simulink model "SF011A_EotLrng"  (R2013b)
settings: Solver=FixedStepDiscrete  SolverMode=SingleTasking  StartTime=0.0  StopTime=1  FixedStep=0.002  RelTol=1e-3
values from neighbouring files (symbols this model uses):
  ARCHGLBPRM_FLOATZEROTHD_ULS_F32 = DataDict.Constant    [SF011A_EotLrng_DataDict.m]
  CNVTOMILLISEC_MILLISECPERCNT_F32 = DataDict.Constant    [SF011A_EotLrng_DataDict.m]
  CORRLNFLT_CNT_U08 = DataDict.Constant    [SF011A_EotLrng_DataDict.m]
  DEBSTEP_CNT_U16 = DataDict.Constant    [SF011A_EotLrng_DataDict.m]
  EOTLIMDETD_CNT_LOGL = DataDict.Constant    [SF011A_EotLrng_DataDict.m]
  EOTLIMNOTDETD_CNT_LOGL = DataDict.Constant    [SF011A_EotLrng_DataDict.m]
  EotLrngAuthyStrtLrn = DataDict.Calibration    [SF011A_EotLrng_DataDict.m]
  EotLrngEotLrnTmr = DataDict.Calibration    [SF011A_EotLrng_DataDict.m]
  EotLrngHwAgOverTrvlCnt = DataDict.Calibration    [SF011A_EotLrng_DataDict.m]
  EotLrngHwAgOverTrvlEntr = DataDict.Calibration    [SF011A_EotLrng_DataDict.m]
  EotLrngHwAgOverTrvlExit = DataDict.Calibration    [SF011A_EotLrng_DataDict.m]
  EotLrngHwTqEotLrn = DataDict.Calibration    [SF011A_EotLrng_DataDict.m]
  EotLrngMotVelEotLrn = DataDict.Calibration    [SF011A_EotLrng_DataDict.m]
  EotLrngRackTrvlMax = DataDict.Calibration    [SF011A_EotLrng_DataDict.m]
  EotLrngRackTrvlMin = DataDict.Calibration    [SF011A_EotLrng_DataDict.m]
  EotLrngRstAuthyMin = DataDict.Calibration    [SF011A_EotLrng_DataDict.m]
  EotProtnRackTrvlLimrEna = DataDict.ImprtdCal    [SF011A_EotLrng_DataDict.m]
  HwAgOverTrvl = DataDict.NTC    [SF011A_EotLrng_DataDict.m]
  HWAGOVERTRVLMAXCNT_CNT_U08 = DataDict.Constant    [SF011A_EotLrng_DataDict.m]
  NODEBSTEP_CNT_U16 = DataDict.Constant    [SF011A_EotLrng_DataDict.m]
  OUTOFRNGFLT_CNT_U08 = DataDict.Constant    [SF011A_EotLrng_DataDict.m]
  RackEotStorgFlt = DataDict.NTC    [SF011A_EotLrng_DataDict.m]
  SIGAVLFLT_CNT_U08 = DataDict.Constant    [SF011A_EotLrng_DataDict.m]
undefined symbols (not defined in the file or in its folder): NtcSts1, NvmGetErrSts1, SigQlfr1
libraries: simulink x19, NxtrNvM x12, NxtrAbslt x5, NxtrLim x4, NxtrMax x3, NxtrMin x3
(part 5 of 7)

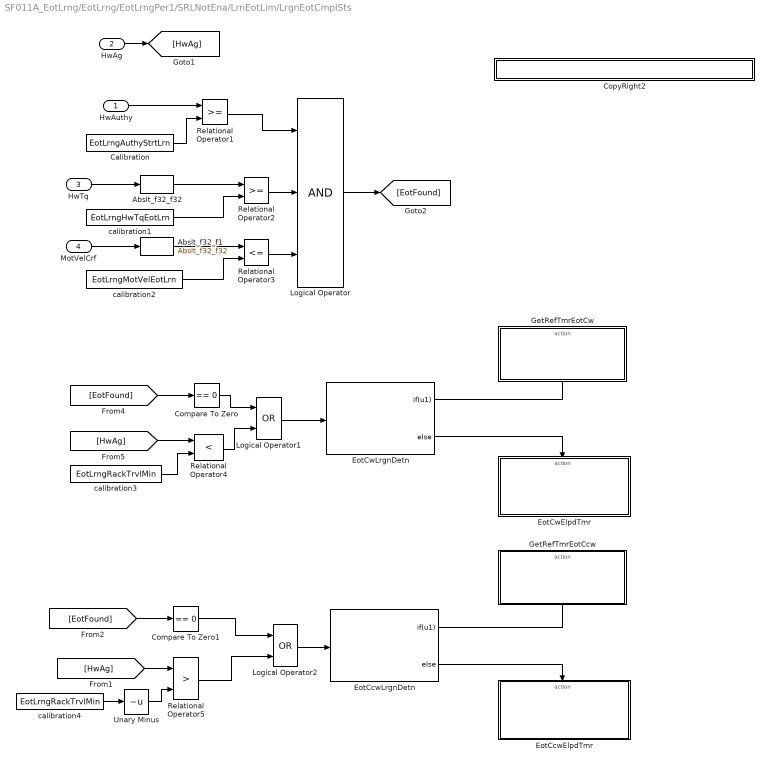
== system SF011A_EotLrng/EotLrng/EotLrngPer1/SRLNotEna/LrnEotLim/LrgnEotCmplSts ==
  HwAuthy : Inport  RequirementInfo="{'linktype_rmi_doors' '0000ba59 (/E-STEER Core/SubSystem Specifications/Application Functions/SF011A Learned EOT Limits)' '#SF011A_137' 'true' 'REQ:  SF011A_137' '' } %GIDa_6ae0917b_799c_4329_b7fc_536c1224b2ae"
  HwAg : Inport  Port=2
  HwTq : Inport  RequirementInfo="{'linktype_rmi_doors' '0000ba59 (/E-STEER Core/SubSystem Specifications/Application Functions/SF011A Learned EOT Limits)' '#SF011A_137' 'true' 'REQ:  SF011A_137' '' } %GIDa_43c992ac_a84d_4c9e_9654_d89dfe1e7ad2"  Port=3
  MotVelCrf : Inport  RequirementInfo="{'linktype_rmi_doors' '0000ba59 (/E-STEER Core/SubSystem Specifications/Application Functions/SF011A Learned EOT Limits)' '#SF011A_137' 'true' 'REQ:  SF011A_137' '' } %GIDa_06bf4615_f553_4b50_9b08_e34adfc1d38a"  Port=4
  Abslt_f32_f1 : NxtrAbslt/Abslt_f32_f32  RequirementInfo="{'linktype_rmi_doors' '0000ba59 (/E-STEER Core/SubSystem Specifications/Application Functions/SF011A Learned EOT Limits)' '#SF011A_137' 'true' 'REQ:  SF011A_137' '' } %GIDa_90d1ac47_d6a5_44ab_bd7c_cda08348b83e"  SFunctionSpec=single y1 = Abslt_f32_f32(single u1)
      settings: AttributesFormatString=%<Name>
  Abslt_f32_f32 : NxtrAbslt/Abslt_f32_f32  RequirementInfo="{'linktype_rmi_doors' '0000ba59 (/E-STEER Core/SubSystem Specifications/Application Functions/SF011A Learned EOT Limits)' '#SF011A_137' 'true' 'REQ:  SF011A_137' '' } %GIDa_6c8d8a4e_2031_40e8_8a2c_4552045f0482"  SFunctionSpec=single y1 = Abslt_f32_f32(single u1)
      settings: AttributesFormatString=%<Name>
  Calibration : Constant  RequirementInfo="{'linktype_rmi_doors' '0000ba59 (/E-STEER Core/SubSystem Specifications/Application Functions/SF011A Learned EOT Limits)' '#SF011A_137' 'true' 'REQ:  SF011A_137' '' } %GIDa_2d58019c_5ecc_462b_8ca1_2e7c37c209ea"  Value=EotLrngAuthyStrtLrn  VectorParams1D=off
  Compare To Zero : simulink/Logic and Bit Operations/Compare To Zero  RequirementInfo="{'linktype_rmi_doors' '0000ba59 (/E-STEER Core/SubSystem Specifications/Application Functions/SF011A Learned EOT Limits)' '#SF011A_138' 'true' 'REQ:  SF011A_138' '' } %GIDa_e7a443f7_7c18_4418_8321_80d1a1d9869a"  relop===  OutDataTypeStr=boolean
  Compare To Zero1 : simulink/Logic and Bit Operations/Compare To Zero  RequirementInfo="{'linktype_rmi_doors' '0000ba59 (/E-STEER Core/SubSystem Specifications/Application Functions/SF011A Learned EOT Limits)' '#SF011A_140' 'true' 'REQ:  SF011A_140' '' } %GIDa_848ff724_1dc5_4b00_8a4d_73899a7f64a0"  relop===  OutDataTypeStr=boolean
  CopyRight2 : Subsystem  Description=|  mask(Copyright Information){none=on}
      | Copyright info block.                                               
      |                                                                     
      | Place copyright information at the top of every subsystem in design.
      mask prompts: none "No parameters"
      mask help: Place copyright information at the top of every subsystem in design.
      mask Display:
      | NxtrConf = 'Nexteer Confidential';
      | 
      | sys = bdroot; %handle for the current model ("system")
      | first = get_param(sys,'Created');
      | if(isempty(first))
      |     first = datestr(now,'yyyy');
      | else
      |     first = first(end-3:end);  %year is last four digits
      | end
      | 
      | last = get_param(sys,'LastModifiedDate');
      | if isempty(last)
      |     last = datestr(now,'yyyy');
      | else
      |     last = last(end-3:end);
      | end
      | 
      | if strcmp(first,last)
      |     fprintf('%s -- Copyright %s Nexteer',NxtrConf,first)
      | else
      |     fprintf('%s -- %s%s- %s Nexteer',NxtrConf,char(169),first,last)
      | end
  EotCcwElpdTmr : Subsystem  TreatAsAtomicUnit=on
  EotCcwLrgnDetn : If  RequirementInfo="{'linktype_rmi_doors' '0000ba59 (/E-STEER Core/SubSystem Specifications/Application Functions/SF011A Learned EOT Limits)' '#SF011A_140' 'true' 'REQ:  SF011A_140' '' } %GIDa_f8f20eef_9892_4bb7_bbd6_f446a50db797"  IfExpression=u1
  EotCwElpdTmr : Subsystem  TreatAsAtomicUnit=on
  EotCwLrgnDetn : If  RequirementInfo="{'linktype_rmi_doors' '0000ba59 (/E-STEER Core/SubSystem Specifications/Application Functions/SF011A Learned EOT Limits)' '#SF011A_138' 'true' 'REQ:  SF011A_138' '' } %GIDa_06ca18a7_da29_4b14_b351_310b9cad5944"  IfExpression=u1
  GetRefTmrEotCcw : Subsystem  RequirementInfo="{'linktype_rmi_doors' '0000ba59 (/E-STEER Core/SubSystem Specifications/Application Functions/SF011A Learned EOT Limits)' '#SF011A_140' 'true' 'REQ:  SF011A_140' '' } %GIDa_8659731a_fa6d_4696_ad55_779c8715d453"  TreatAsAtomicUnit=on
  GetRefTmrEotCw : Subsystem  RequirementInfo="{'linktype_rmi_doors' '0000ba59 (/E-STEER Core/SubSystem Specifications/Application Functions/SF011A Learned EOT Limits)' '#SF011A_138' 'true' 'REQ:  SF011A_138' '' } %GIDa_a6110ea0_4bd3_4935_b54f_86113fc0aff1"  TreatAsAtomicUnit=on
  Logical Operator : Logic  RequirementInfo="{'linktype_rmi_doors' '0000ba59 (/E-STEER Core/SubSystem Specifications/Application Functions/SF011A Learned EOT Limits)' '#SF011A_137' 'true' 'REQ:  SF011A_137' '' } %GIDa_88d5fde5_860a_4825_917f_dc7e0b60601f"  Inputs=3  AllPortsSameDT=off  OutDataTypeStr=boolean
  Logical Operator1 : Logic  RequirementInfo="{'linktype_rmi_doors' '0000ba59 (/E-STEER Core/SubSystem Specifications/Application Functions/SF011A Learned EOT Limits)' '#SF011A_138' 'true' 'REQ:  SF011A_138' '' } %GIDa_3e0f26db_0c97_435b_b6d3_81851007ce5d"  Operator=OR  AllPortsSameDT=off  OutDataTypeStr=boolean
  Logical Operator2 : Logic  RequirementInfo="{'linktype_rmi_doors' '0000ba59 (/E-STEER Core/SubSystem Specifications/Application Functions/SF011A Learned EOT Limits)' '#SF011A_140' 'true' 'REQ:  SF011A_140' '' } %GIDa_49b70cad_20c2_401f_afe8_fdbdd6644c58"  Operator=OR  AllPortsSameDT=off  OutDataTypeStr=boolean
  Relational Operator1 : RelationalOperator  RequirementInfo="{'linktype_rmi_doors' '0000ba59 (/E-STEER Core/SubSystem Specifications/Application Functions/SF011A Learned EOT Limits)' '#SF011A_137' 'true' 'REQ:  SF011A_137' '' } %GIDa_df26607c_7918_4000_898b_821afb5c5f8f"  OutDataTypeStr=boolean
  Relational Operator2 : RelationalOperator  RequirementInfo="{'linktype_rmi_doors' '0000ba59 (/E-STEER Core/SubSystem Specifications/Application Functions/SF011A Learned EOT Limits)' '#SF011A_137' 'true' 'REQ:  SF011A_137' '' } %GIDa_31169408_dc63_4d35_a77a_e15844a3a72e"  OutDataTypeStr=boolean
  Relational Operator3 : RelationalOperator  RequirementInfo="{'linktype_rmi_doors' '0000ba59 (/E-STEER Core/SubSystem Specifications/Application Functions/SF011A Learned EOT Limits)' '#SF011A_137' 'true' 'REQ:  SF011A_137' '' } %GIDa_554488cd_449f_457c_a8f9_9808eaed266b"  Operator=<=  OutDataTypeStr=boolean
  Relational Operator4 : RelationalOperator  RequirementInfo="{'linktype_rmi_doors' '0000ba59 (/E-STEER Core/SubSystem Specifications/Application Functions/SF011A Learned EOT Limits)' '#SF011A_138' 'true' 'REQ:  SF011A_138' '' } %GIDa_8f1b9bdd_eab3_40e5_81ba_aa6e9d80b955"  Operator=<  OutDataTypeStr=boolean
  Relational Operator5 : RelationalOperator  RequirementInfo="{'linktype_rmi_doors' '0000ba59 (/E-STEER Core/SubSystem Specifications/Application Functions/SF011A Learned EOT Limits)' '#SF011A_140' 'true' 'REQ:  SF011A_140' '' } %GIDa_70463160_a2ed_45da_8c6f_b07307a1ab83"  Operator=>  OutDataTypeStr=boolean
  Unary Minus : UnaryMinus  RequirementInfo="{'linktype_rmi_doors' '0000ba59 (/E-STEER Core/SubSystem Specifications/Application Functions/SF011A Learned EOT Limits)' '#SF011A_140' 'true' 'REQ:  SF011A_140' '' } %GIDa_9d4e82f8_ba99_4594_a5e0_a67e1ae72cfe"
  calibration1 : Constant  RequirementInfo="{'linktype_rmi_doors' '0000ba59 (/E-STEER Core/SubSystem Specifications/Application Functions/SF011A Learned EOT Limits)' '#SF011A_137' 'true' 'REQ:  SF011A_137' '' } %GIDa_3c6ef285_bf11_47f3_b917_d6b049015a5b"  Value=EotLrngHwTqEotLrn
  calibration2 : Constant  RequirementInfo="{'linktype_rmi_doors' '0000ba59 (/E-STEER Core/SubSystem Specifications/Application Functions/SF011A Learned EOT Limits)' '#SF011A_137' 'true' 'REQ:  SF011A_137' '' } %GIDa_10c4e04e_7f00_4fce_9c81_2909dc4df01b"  Value=EotLrngMotVelEotLrn
  calibration3 : Constant  RequirementInfo="{'linktype_rmi_doors' '0000ba59 (/E-STEER Core/SubSystem Specifications/Application Functions/SF011A Learned EOT Limits)' '#SF011A_138' 'true' 'REQ:  SF011A_138' '' } %GIDa_030329d4_bb7f_47d8_8321_3bbfe8993bd4"  Value=EotLrngRackTrvlMin
  calibration4 : Constant  RequirementInfo="{'linktype_rmi_doors' '0000ba59 (/E-STEER Core/SubSystem Specifications/Application Functions/SF011A Learned EOT Limits)' '#SF011A_140' 'true' 'REQ:  SF011A_140' '' } %GIDa_70d65ec2_1f3f_4ba7_a4b6_540156069639"  Value=EotLrngRackTrvlMin
  wires:
  EotCwLrgnDetn/2 -> EotCwElpdTmr/Action
  calibration4/1 -> Unary Minus/1
  [HwAg] -> Relational Operator5/1
  HwAuthy/1 -> Relational Operator1/1
  Calibration/1 -> Relational Operator1/2
  Relational Operator5/1 -> Logical Operator2/2
  Abslt_f32_f32/1 -> Relational Operator2/1
  calibration1/1 -> Relational Operator2/2
  Abslt_f32_f1/1 -> Relational Operator3/1
  Relational Operator2/1 -> Logical Operator/2
  calibration2/1 -> Relational Operator3/2
  HwTq/1 -> Abslt_f32_f32/1
  Relational Operator3/1 -> Logical Operator/3
  Logical Operator/1 -> [EotFound]
  MotVelCrf/1 -> Abslt_f32_f1/1
  EotCwLrgnDetn/1 -> GetRefTmrEotCw/Action
  [EotFound] -> Compare To Zero/1
  Logical Operator1/1 -> EotCwLrgnDetn/1
  Relational Operator4/1 -> Logical Operator1/2
  Unary Minus/1 -> Relational Operator5/2
  calibration3/1 -> Relational Operator4/2
  Relational Operator1/1 -> Logical Operator/1
  HwAg/1 -> [HwAg]
  [HwAg] -> Relational Operator4/1
  Compare To Zero/1 -> Logical Operator1/1
  [EotFound] -> Compare To Zero1/1
  Compare To Zero1/1 -> Logical Operator2/1
  Logical Operator2/1 -> EotCcwLrgnDetn/1
  EotCcwLrgnDetn/2 -> EotCcwElpdTmr/Action
  EotCcwLrgnDetn/1 -> GetRefTmrEotCcw/Action

== system SF011A_EotLrng/EotLrng/EotLrngPer1/SRLNotEna/LrnEotLim/LrngEotLim ==
  HwAuthy : Inport  RequirementInfo="{'linktype_rmi_doors' '0000ba59 (/E-STEER Core/SubSystem Specifications/Application Functions/SF011A Learned EOT Limits)' '#SF011A_129' 'true' 'REQ:  SF011A_129' '' } %GIDa_8e9ac969_34cd_4a58_870a_7293dc0412af"
  HwAg : Inport  RequirementInfo="{'linktype_rmi_doors' '0000ba59 (/E-STEER Core/SubSystem Specifications/Application Functions/SF011A Learned EOT Limits)' '#SF011A_129' 'true' 'REQ:  SF011A_129' '' } %GIDa_fc74c770_8175_4ca1_aba5_f58d70c917a2"  Port=2
  Calibration : Constant  RequirementInfo="{'linktype_rmi_doors' '0000ba59 (/E-STEER Core/SubSystem Specifications/Application Functions/SF011A Learned EOT Limits)' '#SF011A_129' 'true' 'REQ:  SF011A_129' '' } %GIDa_f45491c4_44f8_4186_81ac_598397ec509c"  Value=EotLrngAuthyStrtLrn
  CmpLim : Subsystem  RequirementInfo="{'linktype_rmi_doors' '0000ba59 (/E-STEER Core/SubSystem Specifications/Application Functions/SF011A Learned EOT Limits)' '#SF011A_129' 'true' 'REQ:  SF011A_129' '' } %GIDa_5796e9fa_2131_4501_9acb_7c4fc47bfd1b"  TreatAsAtomicUnit=on
  CopyRight2 : Subsystem  Description=|  mask(Copyright Information){none=on}
      | Copyright info block.                                               
      |                                                                     
      | Place copyright information at the top of every subsystem in design.
      mask prompts: none "No parameters"
      mask help: Place copyright information at the top of every subsystem in design.
      mask Display:
      | NxtrConf = 'Nexteer Confidential';
      | 
      | sys = bdroot; %handle for the current model ("system")
      | first = get_param(sys,'Created');
      | if(isempty(first))
      |     first = datestr(now,'yyyy');
      | else
      |     first = first(end-3:end);  %year is last four digits
      | end
      | 
      | last = get_param(sys,'LastModifiedDate');
      | if isempty(last)
      |     last = datestr(now,'yyyy');
      | else
      |     last = last(end-3:end);
      | end
      | 
      | if strcmp(first,last)
      |     fprintf('%s -- Copyright %s Nexteer',NxtrConf,first)
      | else
      |     fprintf('%s -- %s%s- %s Nexteer',NxtrConf,char(169),first,last)
      | end
  If : If  RequirementInfo="{'linktype_rmi_doors' '0000ba59 (/E-STEER Core/SubSystem Specifications/Application Functions/SF011A Learned EOT Limits)' '#SF011A_129' 'true' 'REQ:  SF011A_129' '' } %GIDa_24c81cd6_03b6_4618_bb0b_3e338bf864c1"  IfExpression=u1  ShowElse=off
  Relational Operator1 : RelationalOperator  RequirementInfo="{'linktype_rmi_doors' '0000ba59 (/E-STEER Core/SubSystem Specifications/Application Functions/SF011A Learned EOT Limits)' '#SF011A_129' 'true' 'REQ:  SF011A_129' '' } %GIDa_dbed88ab_8929_485e_9400_c10456725ed5"  OutDataTypeStr=boolean
  wires:
  HwAg/1 -> CmpLim/1(HwAg)
  If/1 -> CmpLim/Action
  Calibration/1 -> Relational Operator1/2
  Relational Operator1/1 -> If/1
  HwAuthy/1 -> Relational Operator1/1

== system SF011A_EotLrng/EotLrng/EotLrngPer1/SRLNotEna/RstEot/ChkRstLimReq ==
  Action Port : ActionPort  ActionType=then
  CopyRight2 : Subsystem  Description=|  mask(Copyright Information){none=on}
      | Copyright info block.                                               
      |                                                                     
      | Place copyright information at the top of every subsystem in design.
      mask prompts: none "No parameters"
      mask help: Place copyright information at the top of every subsystem in design.
      mask Display:
      | NxtrConf = 'Nexteer Confidential';
      | 
      | sys = bdroot; %handle for the current model ("system")
      | first = get_param(sys,'Created');
      | if(isempty(first))
      |     first = datestr(now,'yyyy');
      | else
      |     first = first(end-3:end);  %year is last four digits
      | end
      | 
      | last = get_param(sys,'LastModifiedDate');
      | if isempty(last)
      |     last = datestr(now,'yyyy');
      | else
      |     last = last(end-3:end);
      | end
      | 
      | if strcmp(first,last)
      |     fprintf('%s -- Copyright %s Nexteer',NxtrConf,first)
      | else
      |     fprintf('%s -- %s%s- %s Nexteer',NxtrConf,char(169),first,last)
      | end
  Data Store Read4 : DataStoreRead  RequirementInfo="{'linktype_rmi_doors' '0000ba59 (/E-STEER Core/SubSystem Specifications/Application Functions/SF011A Learned EOT Limits)' '#SF011A_120' 'true' 'REQ:  SF011A_120' '' } %GIDa_cfa4e016_6ae4_4862_9550_c74d96b3c73b"  DataStoreName=RstLimReq
  If : If  RequirementInfo="{'linktype_rmi_doors' '0000ba59 (/E-STEER Core/SubSystem Specifications/Application Functions/SF011A Learned EOT Limits)' '#SF011A_120' 'true' 'REQ:  SF011A_120' '' } %GIDa_773e02fb_f8a3_4af3_8112_ebd8a98039fa"  IfExpression=u1  ShowElse=off
  ResetLimReq : Subsystem  RequirementInfo="{'linktype_rmi_doors' '0000ba59 (/E-STEER Core/SubSystem Specifications/Application Functions/SF011A Learned EOT Limits)' '#SF011A_120' 'true' 'REQ:  SF011A_120' '' } %GIDa_bb201849_3e58_4b73_888b_0620fb1d4089"  TreatAsAtomicUnit=on
  wires:
  Data Store Read4/1 -> If/1
  If/1 -> ResetLimReq/Action

== system SF011A_EotLrng/EotLrng/EotLrngPer1/SRLNotEna/RstEot/Copyright1 ==

== system SF011A_EotLrng/EotLrng/EotLrngInit1/RstEot/ChkRstLimReq/ResetLimReq/Copyright1 ==

== system SF011A_EotLrng/EotLrng/EotLrngPer1/HwAgCwAndCcwMax/HwAgCwAndCcw/MaxHwAgCcwDetd/CopyRight2 ==

== system SF011A_EotLrng/EotLrng/EotLrngPer1/HwAgCwAndCcwMax/HwAgCwAndCcw/MaxHwAgCwDetd/CopyRight2 ==

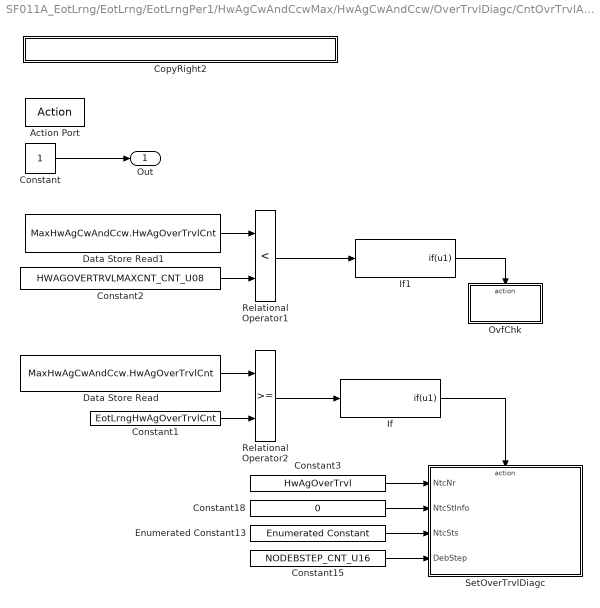
== system SF011A_EotLrng/EotLrng/EotLrngPer1/HwAgCwAndCcwMax/HwAgCwAndCcw/OverTrvlDiagc/CntOvrTrvlAndSetNTC ==
  Action Port : ActionPort  ActionType=then
  Constant : Constant  OutDataTypeStr=boolean
      settings: AttributesFormatString=%<OutDataTypeStr>
  Constant1 : Constant  RequirementInfo="{'linktype_rmi_doors' '0000ba59 (/E-STEER Core/SubSystem Specifications/Application Functions/SF011A Learned EOT Limits)' '#SF011A_208' 'true' 'REQ:  SF011A_208' '' } %GIDa_75f3c349_1807_46d6_9a05_a47c9f2917b5"  Value=EotLrngHwAgOverTrvlCnt
  Constant15 : Constant  RequirementInfo={} %GIDa_ff38e660_0bb6_4878_9217_21f6e62faf0b  Value=NODEBSTEP_CNT_U16
  Constant18 : Constant  RequirementInfo={} %GIDa_47badf73_4199_4dd3_af71_217d29069f8a  Value=0
  Constant2 : Constant  Value=HWAGOVERTRVLMAXCNT_CNT_U08  OutDataTypeStr=uint8
      settings: AttributesFormatString=%<OutDataTypeStr>
  Constant3 : Constant  RequirementInfo={} %GIDa_975f3d12_92c7_415c_a670_86e9a0b5cae7  Value=HwAgOverTrvl
  CopyRight2 : Subsystem  Description=|  mask(Copyright Information){none=on}
      | Copyright info block.                                               
      |                                                                     
      | Place copyright information at the top of every subsystem in design.
      mask prompts: none "No parameters"
      mask help: Place copyright information at the top of every subsystem in design.
      mask Display:
      | NxtrConf = 'Nexteer Confidential';
      | 
      | sys = bdroot; %handle for the current model ("system")
      | first = get_param(sys,'Created');
      | if(isempty(first))
      |     first = datestr(now,'yyyy');
      | else
      |     first = first(end-3:end);  %year is last four digits
      | end
      | 
      | last = get_param(sys,'LastModifiedDate');
      | if isempty(last)
      |     last = datestr(now,'yyyy');
      | else
      |     last = last(end-3:end);
      | end
      | 
      | if strcmp(first,last)
      |     fprintf('%s -- Copyright %s Nexteer',NxtrConf,first)
      | else
      |     fprintf('%s -- %s%s- %s Nexteer',NxtrConf,char(169),first,last)
      | end
  Data Store Read : DataStoreRead  RequirementInfo="{'linktype_rmi_doors' '0000ba59 (/E-STEER Core/SubSystem Specifications/Application Functions/SF011A Learned EOT Limits)' '#SF011A_208' 'true' 'REQ:  SF011A_208' '' } %GIDa_b4a55bbd_2227_4382_a31b_8a234d8b9da7"  DataStoreName=MaxHwAgCwAndCcw  DataStoreElements=MaxHwAgCwAndCcw.HwAgOverTrvlCnt
  Data Store Read1 : DataStoreRead  DataStoreName=MaxHwAgCwAndCcw  DataStoreElements=MaxHwAgCwAndCcw.HwAgOverTrvlCnt
  Enumerated Constant13 : simulink/Sources/Enumerated Constant  RequirementInfo={} %GIDa_1bc7ccae_3244_4a0b_af3a_7db8881d82ae  OutDataTypeStr=Enum: NtcSts1  Value=NtcSts1.NTCSTS_FAILD  SampleTime=inf
  If : If  RequirementInfo="{'linktype_rmi_doors' '0000ba59 (/E-STEER Core/SubSystem Specifications/Application Functions/SF011A Learned EOT Limits)' '#SF011A_208' 'true' 'REQ:  SF011A_208' '' } %GIDa_3e7dc2dc_2377_4dcd_b250_0a8fc5b27089"  Priority=1  IfExpression=u1  ShowElse=off
      settings: AttributesFormatString=Priority = %<Priority>
  If1 : If  Priority=0  IfExpression=u1  ShowElse=off
      settings: AttributesFormatString=Priority = %<Priority>
  OvfChk : Subsystem  RequirementInfo="{'linktype_rmi_doors' '0000ba59 (/E-STEER Core/SubSystem Specifications/Application Functions/SF011A Learned EOT Limits)' '#SF011A_183' 'true' 'REQ:  SF011A_183' '' ; 'linktype_rmi_doors' '0000ba59 (/E-STEER Core/SubSystem Specifications/Application Functions/SF011A Learned EOT Limits)' '#SF011A_176' 'true' 'REQ:  SF011A_176' '' } %GIDa_08e64fd8_f2e0_4d32_8256_5fd2dd45fe7b"  TreatAsAtomicUnit=on
  Relational Operator1 : RelationalOperator  RequirementInfo={} %GIDa_2b1f267d_7ae5_42af_952d_58a478c3f374  Operator=<  OutDataTypeStr=boolean
  Relational Operator2 : RelationalOperator  RequirementInfo="{'linktype_rmi_doors' '0000ba59 (/E-STEER Core/SubSystem Specifications/Application Functions/SF011A Learned EOT Limits)' '#SF011A_208' 'true' 'REQ:  SF011A_208' '' } %GIDa_4b5efb5d_37c5_4623_83be_764c5aa43908"  OutDataTypeStr=boolean
  SetOverTrvlDiagc : Subsystem  RequirementInfo="{'linktype_rmi_doors' '0000ba59 (/E-STEER Core/SubSystem Specifications/Application Functions/SF011A Learned EOT Limits)' '#SF011A_208' 'true' 'REQ:  SF011A_208' '' } %GIDa_fe30b093_ba03_4d28_8071_2fbc9853f1a8"  mask(SetNTC){}
      mask help: SetNTC library block
  Out : Outport
  wires:
  Constant1/1 -> Relational Operator2/2
  Relational Operator2/1 -> If/1
  If/1 -> SetOverTrvlDiagc/Action
  Constant15/1 -> SetOverTrvlDiagc/4(DebStep)
  Enumerated Constant13/1 -> SetOverTrvlDiagc/3(NtcSts)
  Constant18/1 -> SetOverTrvlDiagc/2(NtcStInfo)
  Constant3/1 -> SetOverTrvlDiagc/1(NtcNr)
  Data Store Read1/1 -> Relational Operator1/1
  Data Store Read/1 -> Relational Operator2/1
  Constant2/1 -> Relational Operator1/2
  Relational Operator1/1 -> If1/1
  If1/1 -> OvfChk/Action
  Constant/1 -> Out/1

== system SF011A_EotLrng/EotLrng/EotLrngPer1/HwAgCwAndCcwMax/HwAgCwAndCcw/OverTrvlDiagc/CopyRight2 ==

== system SF011A_EotLrng/EotLrng/EotLrngPer1/HwAgCwAndCcwMax/HwAgCwAndCcw/OverTrvlDiagc/HwAgEntrCdn ==
  HwAg : Inport
  Constant1 : Constant  Value=EotLrngHwAgOverTrvlEntr
  CopyRight2 : Subsystem  Description=|  mask(Copyright Information){none=on}
      | Copyright info block.                                               
      |                                                                     
      | Place copyright information at the top of every subsystem in design.
      mask prompts: none "No parameters"
      mask help: Place copyright information at the top of every subsystem in design.
      mask Display:
      | NxtrConf = 'Nexteer Confidential';
      | 
      | sys = bdroot; %handle for the current model ("system")
      | first = get_param(sys,'Created');
      | if(isempty(first))
      |     first = datestr(now,'yyyy');
      | else
      |     first = first(end-3:end);  %year is last four digits
      | end
      | 
      | last = get_param(sys,'LastModifiedDate');
      | if isempty(last)
      |     last = datestr(now,'yyyy');
      | else
      |     last = last(end-3:end);
      | end
      | 
      | if strcmp(first,last)
      |     fprintf('%s -- Copyright %s Nexteer',NxtrConf,first)
      | else
      |     fprintf('%s -- %s%s- %s Nexteer',NxtrConf,char(169),first,last)
      | end
  Relational Operator2 : RelationalOperator  RequirementInfo={} %GIDa_009d59f0_7f21_4d15_bb28_332f54a9bb97  Operator=>  OutDataTypeStr=boolean
  Out : Outport
  wires:
  Relational Operator2/1 -> Out/1
  HwAg/1 -> Relational Operator2/1
  Constant1/1 -> Relational Operator2/2

== system SF011A_EotLrng/EotLrng/EotLrngPer1/HwAgCwAndCcwMax/HwAgCwAndCcw/OverTrvlDiagc/HwAgExitCdn ==
  HwAg : Inport
  Constant1 : Constant  Value=EotLrngHwAgOverTrvlExit
  CopyRight2 : Subsystem  Description=|  mask(Copyright Information){none=on}
      | Copyright info block.                                               
      |                                                                     
      | Place copyright information at the top of every subsystem in design.
      mask prompts: none "No parameters"
      mask help: Place copyright information at the top of every subsystem in design.
      mask Display:
      | NxtrConf = 'Nexteer Confidential';
      | 
      | sys = bdroot; %handle for the current model ("system")
      | first = get_param(sys,'Created');
      | if(isempty(first))
      |     first = datestr(now,'yyyy');
      | else
      |     first = first(end-3:end);  %year is last four digits
      | end
      | 
      | last = get_param(sys,'LastModifiedDate');
      | if isempty(last)
      |     last = datestr(now,'yyyy');
      | else
      |     last = last(end-3:end);
      | end
      | 
      | if strcmp(first,last)
      |     fprintf('%s -- Copyright %s Nexteer',NxtrConf,first)
      | else
      |     fprintf('%s -- %s%s- %s Nexteer',NxtrConf,char(169),first,last)
      | end
  Relational Operator2 : RelationalOperator  RequirementInfo={} %GIDa_2c1adbcd_f9bd_463a_a4ba_4deb565835e8  Operator=<  OutDataTypeStr=boolean
  Out : Outport
  wires:
  Relational Operator2/1 -> Out/1
  Constant1/1 -> Relational Operator2/2
  HwAg/1 -> Relational Operator2/1

== system SF011A_EotLrng/EotLrng/EotLrngPer1/HwAgCwAndCcwMax/HwAgCwAndCcw/OverTrvlDiagc/Pass ==
  Action Port : ActionPort  ActionType=else
  " " : DataStoreRead  DataStoreName=HwAgOverTrvlCntrDi
  CopyRight2 : Subsystem  Description=|  mask(Copyright Information){none=on}
      | Copyright info block.                                               
      |                                                                     
      | Place copyright information at the top of every subsystem in design.
      mask prompts: none "No parameters"
      mask help: Place copyright information at the top of every subsystem in design.
      mask Display:
      | NxtrConf = 'Nexteer Confidential';
      | 
      | sys = bdroot; %handle for the current model ("system")
      | first = get_param(sys,'Created');
      | if(isempty(first))
      |     first = datestr(now,'yyyy');
      | else
      |     first = first(end-3:end);  %year is last four digits
      | end
      | 
      | last = get_param(sys,'LastModifiedDate');
      | if isempty(last)
      |     last = datestr(now,'yyyy');
      | else
      |     last = last(end-3:end);
      | end
      | 
      | if strcmp(first,last)
      |     fprintf('%s -- Copyright %s Nexteer',NxtrConf,first)
      | else
      |     fprintf('%s -- %s%s- %s Nexteer',NxtrConf,char(169),first,last)
      | end
  Out : Outport
  wires:
  " "/1 -> Out/1

== system SF011A_EotLrng/EotLrng/EotLrngPer1/HwAgCwAndCcwMax/HwAgCwAndCcw/OverTrvlDiagc/RstHwAgOverTrvlSwtVari ==
  Action Port : ActionPort  ActionType=elseif
  " " : Constant  Value=0  OutDataTypeStr=boolean  LockScale=on
      settings: AttributesFormatString=%<OutDataTypeStr>
  CopyRight2 : Subsystem  Description=|  mask(Copyright Information){none=on}
      | Copyright info block.                                               
      |                                                                     
      | Place copyright information at the top of every subsystem in design.
      mask prompts: none "No parameters"
      mask help: Place copyright information at the top of every subsystem in design.
      mask Display:
      | NxtrConf = 'Nexteer Confidential';
      | 
      | sys = bdroot; %handle for the current model ("system")
      | first = get_param(sys,'Created');
      | if(isempty(first))
      |     first = datestr(now,'yyyy');
      | else
      |     first = first(end-3:end);  %year is last four digits
      | end
      | 
      | last = get_param(sys,'LastModifiedDate');
      | if isempty(last)
      |     last = datestr(now,'yyyy');
      | else
      |     last = last(end-3:end);
      | end
      | 
      | if strcmp(first,last)
      |     fprintf('%s -- Copyright %s Nexteer',NxtrConf,first)
      | else
      |     fprintf('%s -- %s%s- %s Nexteer',NxtrConf,char(169),first,last)
      | end
  Out : Outport
  wires:
  " "/1 -> Out/1

== system SF011A_EotLrng/EotLrng/EotLrngPer1/SRLEna/ChkEotSigForNtc/EotSigAvl/CopyRight2 ==

== system SF011A_EotLrng/EotLrng/EotLrngPer1/SRLEna/ChkEotSigForNtc/EotSigAvl/SetCorrlFltNtc ==
  NtcNr : Inport
  NtcStInfo : Inport  Port=2
  NtcSts : Inport  Port=3
  DebStep : Inport  Port=4
  CallDiagMgr : ActionPort  ActionType=elseif
  SetNtcSts : Subsystem  RequirementInfo={} %GIDa_64273598_829f_4830_91ff_4cc9249c356b  TreatAsAtomicUnit=on
      settings: RTWSystemCode=Inline
  wires:
  NtcNr/1 -> SetNtcSts/1(NtcNr)  "NtcNr"
  NtcSts/1 -> SetNtcSts/3(NtcSts)
  DebStep/1 -> SetNtcSts/4(DebStep)
  NtcStInfo/1 -> SetNtcSts/2(NtcStInfo)

== system SF011A_EotLrng/EotLrng/EotLrngPer1/SRLEna/ChkEotSigForNtc/EotSigAvl/SetOutOfRngNtc ==
  NtcNr : Inport
  NtcStInfo : Inport  Port=2
  NtcSts : Inport  Port=3
  DebStep : Inport  Port=4
  CallDiagMgr : ActionPort  ActionType=else
  SetNtcSts : Subsystem  RequirementInfo={} %GIDa_969e9bed_97c2_4412_864b_301db2fcd816  TreatAsAtomicUnit=on
      settings: RTWSystemCode=Inline
  wires:
  NtcStInfo/1 -> SetNtcSts/2(NtcStInfo)
  DebStep/1 -> SetNtcSts/4(DebStep)
  NtcSts/1 -> SetNtcSts/3(NtcSts)
  NtcNr/1 -> SetNtcSts/1(NtcNr)  "NtcNr"

== system SF011A_EotLrng/EotLrng/EotLrngPer1/SRLEna/ChkEotSigForNtc/EotSigAvl/Update NVM ==
  EotSig0Cw : Inport  RequirementInfo="{'linktype_rmi_doors' '0000ba59 (/E-STEER Core/SubSystem Specifications/Application Functions/SF011A Learned EOT Limits)' '#SF011A_145' 'true' 'REQ:  SF011A_145' '' } %GIDa_daca1601_86a1_4488_9c8e_d2e3970afb9b"
  EotSig0Ccw : Inport  RequirementInfo="{'linktype_rmi_doors' '0000ba59 (/E-STEER Core/SubSystem Specifications/Application Functions/SF011A Learned EOT Limits)' '#SF011A_145' 'true' 'REQ:  SF011A_145' '' } %GIDa_f3269ded_08ac_421a_8638_6305717386f0"  Port=2
  Action Port : ActionPort  ActionType=then
  CcwDetdFlag : Constant  RequirementInfo="{'linktype_rmi_doors' '0000ba59 (/E-STEER Core/SubSystem Specifications/Application Functions/SF011A Learned EOT Limits)' '#SF011A_145' 'true' 'REQ:  SF011A_145' '' } %GIDa_69bcb2fc_dcfb_4055_8819_d39dee54556b"  Value=EOTLIMDETD_CNT_LOGL
  Constant1 : Constant  RequirementInfo="{'linktype_rmi_doors' '0000ba59 (/E-STEER Core/SubSystem Specifications/Application Functions/SF011A Learned EOT Limits)' '#SF011A_145' 'true' 'REQ:  SF011A_145' '' ; 'linktype_rmi_doors' '0000ba59 (/E-STEER Core/SubSystem Specifications/Application Functions/SF011A Learned EOT Limits)' '#SF011A_165' 'true' 'REQ:  SF011A_165' '' } %GIDa_eb6d3d4c_31f5_4c7e_849f_3b94922d4e6f"  Value=RackEotStorgFlt
  Constant15 : Constant  RequirementInfo="{'linktype_rmi_doors' '0000ba59 (/E-STEER Core/SubSystem Specifications/Application Functions/SF011A Learned EOT Limits)' '#SF011A_145' 'true' 'REQ:  SF011A_145' '' ; 'linktype_rmi_doors' '0000ba59 (/E-STEER Core/SubSystem Specifications/Application Functions/SF011A Learned EOT Limits)' '#SF011A_165' 'true' 'REQ:  SF011A_165' '' } %GIDa_ee551ea2_91a8_4a4b_8ecb_101194a42d12"  Value=NODEBSTEP_CNT_U16
  Constant18 : Constant  RequirementInfo="{'linktype_rmi_doors' '0000ba59 (/E-STEER Core/SubSystem Specifications/Application Functions/SF011A Learned EOT Limits)' '#SF011A_145' 'true' 'REQ:  SF011A_145' '' ; 'linktype_rmi_doors' '0000ba59 (/E-STEER Core/SubSystem Specifications/Application Functions/SF011A Learned EOT Limits)' '#SF011A_165' 'true' 'REQ:  SF011A_165' '' } %GIDa_6273788d_273f_4442_a88c_8c3ffb566926"  Value=0
  CopyRight2 : Subsystem  Description=|  mask(Copyright Information){none=on}
      | Copyright info block.                                               
      |                                                                     
      | Place copyright information at the top of every subsystem in design.
      mask prompts: none "No parameters"
      mask help: Place copyright information at the top of every subsystem in design.
      mask Display:
      | NxtrConf = 'Nexteer Confidential';
      | 
      | sys = bdroot; %handle for the current model ("system")
      | first = get_param(sys,'Created');
      | if(isempty(first))
      |     first = datestr(now,'yyyy');
      | else
      |     first = first(end-3:end);  %year is last four digits
      | end
      | 
      | last = get_param(sys,'LastModifiedDate');
      | if isempty(last)
      |     last = datestr(now,'yyyy');
      | else
      |     last = last(end-3:end);
      | end
      | 
      | if strcmp(first,last)
      |     fprintf('%s -- Copyright %s Nexteer',NxtrConf,first)
      | else
      |     fprintf('%s -- %s%s- %s Nexteer',NxtrConf,char(169),first,last)
      | end
  CwDetdFlag : Constant  RequirementInfo="{'linktype_rmi_doors' '0000ba59 (/E-STEER Core/SubSystem Specifications/Application Functions/SF011A Learned EOT Limits)' '#SF011A_145' 'true' 'REQ:  SF011A_145' '' } %GIDa_efcee59d_77f5_4767_b53e_457262cca54c"  Value=EOTLIMDETD_CNT_LOGL
  Enumerated Constant13 : simulink/Sources/Enumerated Constant  RequirementInfo="{'linktype_rmi_doors' '0000ba59 (/E-STEER Core/SubSystem Specifications/Application Functions/SF011A Learned EOT Limits)' '#SF011A_145' 'true' 'REQ:  SF011A_145' '' ; 'linktype_rmi_doors' '0000ba59 (/E-STEER Core/SubSystem Specifications/Application Functions/SF011A Learned EOT Limits)' '#SF011A_165' 'true' 'REQ:  SF011A_165' '' } %GIDa_876016d1_f5a9_4bda_a276_91c8da69ecbf"  OutDataTypeStr=Enum: NtcSts1  Value=NtcSts1.NTCSTS_PASSD  SampleTime=inf
  Set Ram Block Status : NxtrNvM/Set Ram Block Status  RequirementInfo="{'linktype_rmi_doors' '0000ba59 (/E-STEER Core/SubSystem Specifications/Application Functions/SF011A Learned EOT Limits)' '#SF011A_156' 'true' 'REQ:  SF011A_156' '' } %GIDa_55d737c2_273c_40b5_868b_e71ef2331b9d"  FuncName=Set Ram Block Status  NvMBlockName=EotNvmdata  VoidFuncRtn=on  BlockChanged_DSN=NvMSRBS_BlockChanged3  Return_DSN=NvMSRBS_Return3
      settings: AttributesFormatString=%<FuncName>
  SetNTCPass : Subsystem  RequirementInfo="{'linktype_rmi_doors' '0000ba59 (/E-STEER Core/SubSystem Specifications/Application Functions/SF011A Learned EOT Limits)' '#SF011A_145' 'true' 'REQ:  SF011A_145' '' ; 'linktype_rmi_doors' '0000ba59 (/E-STEER Core/SubSystem Specifications/Application Functions/SF011A Learned EOT Limits)' '#SF011A_165' 'true' 'REQ:  SF011A_165' '' } %GIDa_c93011ea_1cec_4e5f_87df_22d47cf632a9"  mask(SetNTC){}
      mask help: SetNTC library block
  Update PIM : DataStoreWrite  RequirementInfo="{'linktype_rmi_doors' '0000ba59 (/E-STEER Core/SubSystem Specifications/Application Functions/SF011A Learned EOT Limits)' '#SF011A_145' 'true' 'REQ:  SF011A_145' '' } %GIDa_963b29fc_65db_4efa_a492_40cbd9360cfc"  DataStoreName=EotNvmData  DataStoreElements=EotNvmData.CwEot#EotNvmData.CcwEot#EotNvmData.CwEotDetd#EotNvmData.CcwEotDetd
  WriteFlag : Constant  RequirementInfo="{'linktype_rmi_doors' '0000ba59 (/E-STEER Core/SubSystem Specifications/Application Functions/SF011A Learned EOT Limits)' '#SF011A_156' 'true' 'REQ:  SF011A_156' '' } %GIDa_5b9cd5d6_0b7d_4b98_b87e_5713c3ded4e6"  OutDataTypeStr=boolean
      settings: AttributesFormatString=%<OutDataTypeStr>
  wires:
  EotSig0Cw/1 -> Update PIM/1
  EotSig0Ccw/1 -> Update PIM/2
  CcwDetdFlag/1 -> Update PIM/4
  CwDetdFlag/1 -> Update PIM/3
  WriteFlag/1 -> Set Ram Block Status/1
  Constant15/1 -> SetNTCPass/4(DebStep)
  Enumerated Constant13/1 -> SetNTCPass/3(NtcSts)
  Constant18/1 -> SetNTCPass/2(NtcStInfo)
  Constant1/1 -> SetNTCPass/1(NtcNr)

== system SF011A_EotLrng/EotLrng/EotLrngPer1/SRLEna/ChkEotSigForNtc/SetSigAvlFltNtc/SetNtcSts ==
  note: Note:
      |
      | - "ISO Fault Debounce Design" Simulink block intent to use here for Simulation purpose only. Do not Code this block
  NtcNr : Inport
  NtcStInfo : Inport  Port=2
  NtcSts : Inport  Port=3
  DebStep : Inport  Port=4
  CopyRight2 : Subsystem  Description=|  mask(Copyright Information){none=on}
      | Copyright info block.                                               
      |                                                                     
      | Place copyright information at the top of every subsystem in design.
      mask prompts: none "No parameters"
      mask help: Place copyright information at the top of every subsystem in design.
      mask Display:
      | NxtrConf = 'Nexteer Confidential';
      | 
      | sys = bdroot; %handle for the current model ("system")
      | first = get_param(sys,'Created');
      | if(isempty(first))
      |     first = datestr(now,'yyyy');
      | else
      |     first = first(end-3:end);  %year is last four digits
      | end
      | 
      | last = get_param(sys,'LastModifiedDate');
      | if isempty(last)
      |     last = datestr(now,'yyyy');
      | else
      |     last = last(end-3:end);
      | end
      | 
      | if strcmp(first,last)
      |     fprintf('%s -- Copyright %s Nexteer',NxtrConf,first)
      | else
      |     fprintf('%s -- %s%s- %s Nexteer',NxtrConf,char(169),first,last)
      | end
  Data Store Write : DataStoreWrite  DataStoreName=NtcQlfr
  Data Store Write1 : DataStoreWrite  DataStoreName=NtcQlfrVal
  Data Store Write2 : DataStoreWrite  DataStoreName=NtcStInfoVal
  Data Store Write3 : DataStoreWrite  DataStoreName=NtcStsVal
  Data Type Conversion : DataTypeConversion  OutDataTypeStr=Enum: SigQlfr1
  Data Type Conversion1 : DataTypeConversion  OutDataTypeStr=uint8
  Ground : Ground
  ISO Fault Debounce Design : Stateflow chart  TreatAsAtomicUnit=on
      settings: AttributesFormatString=|
      | Simulation Purpose Only.
      | Do Not Code this block
      | Diagnostic Manager Owns this requirement
  Terminator : Terminator
  Terminator1 : Terminator
  wires:
  NtcNr/1 -> Terminator/1
  DebStep/1 -> ISO Fault Debounce Design/2(DebStep)
  ISO Fault Debounce Design/1(Qualifier) -> Data Type Conversion/1
  Ground/1 -> ISO Fault Debounce Design/3(SvcClr)
  NtcSts/1 -> Data Store Write3/1, ISO Fault Debounce Design/1(NtcSts)
  Data Type Conversion/1 -> Data Store Write1/1, Data Store Write/1
  NtcStInfo/1 -> Data Type Conversion1/1, Terminator1/1
  Data Type Conversion1/1 -> Data Store Write2/1

== system SF011A_EotLrng/EotLrng/EotLrngPer1/SRLNotEna/LrnEotLim/LrgnEotCmplSts/CopyRight2 ==

== system SF011A_EotLrng/EotLrng/EotLrngPer1/SRLNotEna/LrnEotLim/LrgnEotCmplSts/EotCcwElpdTmr ==
  Action Port : ActionPort  ActionType=else
  CopyRight2 : Subsystem  Description=|  mask(Copyright Information){none=on}
      | Copyright info block.                                               
      |                                                                     
      | Place copyright information at the top of every subsystem in design.
      mask prompts: none "No parameters"
      mask help: Place copyright information at the top of every subsystem in design.
      mask Display:
      | NxtrConf = 'Nexteer Confidential';
      | 
      | sys = bdroot; %handle for the current model ("system")
      | first = get_param(sys,'Created');
      | if(isempty(first))
      |     first = datestr(now,'yyyy');
      | else
      |     first = first(end-3:end);  %year is last four digits
      | end
      | 
      | last = get_param(sys,'LastModifiedDate');
      | if isempty(last)
      |     last = datestr(now,'yyyy');
      | else
      |     last = last(end-3:end);
      | end
      | 
      | if strcmp(first,last)
      |     fprintf('%s -- Copyright %s Nexteer',NxtrConf,first)
      | else
      |     fprintf('%s -- %s%s- %s Nexteer',NxtrConf,char(169),first,last)
      | end
  Data Store Read1 : DataStoreRead  RequirementInfo="{'linktype_rmi_doors' '0000ba59 (/E-STEER Core/SubSystem Specifications/Application Functions/SF011A Learned EOT Limits)' '#SF011A_141' 'true' 'REQ:  SF011A_141' '' } %GIDa_c03cce4d_3eed_45ef_9fa3_207aeb1d770f"  DataStoreName=CcwEotRefTmr
  Divide2 : Product  RequirementInfo="{'linktype_rmi_doors' '0000ba59 (/E-STEER Core/SubSystem Specifications/Application Functions/SF011A Learned EOT Limits)' '#SF011A_141' 'true' 'REQ:  SF011A_141' '' } %GIDa_da988bbf_3003_4036_ae14_57d6b2f38e17"  Inputs=**
  EotCcwLrgnDetd : Subsystem  RequirementInfo="{'linktype_rmi_doors' '0000ba59 (/E-STEER Core/SubSystem Specifications/Application Functions/SF011A Learned EOT Limits)' '#SF011A_141' 'true' 'REQ:  SF011A_141' '' } %GIDa_fb71c179_1321_4c80_92b7_944c6f3576c7"  TreatAsAtomicUnit=on
  GetTiSpan100MicroSec32bit : Subsystem  mask(Timer_GTS){}
      mask help: Used to get the time span between start and current time.
  MillisecPerCount : Constant  RequirementInfo="{'linktype_rmi_doors' '0000ba59 (/E-STEER Core/SubSystem Specifications/Application Functions/SF011A Learned EOT Limits)' '#SF011A_141' 'true' 'REQ:  SF011A_141' '' } %GIDa_df556f57_2489_40d0_91ed_1a4ad46fc88f"  Value=CNVTOMILLISEC_MILLISECPERCNT_F32
  Relational Operator1 : RelationalOperator  RequirementInfo="{'linktype_rmi_doors' '0000ba59 (/E-STEER Core/SubSystem Specifications/Application Functions/SF011A Learned EOT Limits)' '#SF011A_141' 'true' 'REQ:  SF011A_141' '' } %GIDa_9b0da4b8_4894_4677_936a_ea8631a97591"  OutDataTypeStr=boolean
  TmrElpdDetn : If  RequirementInfo="{'linktype_rmi_doors' '0000ba59 (/E-STEER Core/SubSystem Specifications/Application Functions/SF011A Learned EOT Limits)' '#SF011A_141' 'true' 'REQ:  SF011A_141' '' } %GIDa_2ee5c93d_4881_40b1_a18b_8bf5a925f407"  IfExpression=u1  ShowElse=off
  calibration6 : Constant  RequirementInfo="{'linktype_rmi_doors' '0000ba59 (/E-STEER Core/SubSystem Specifications/Application Functions/SF011A Learned EOT Limits)' '#SF011A_141' 'true' 'REQ:  SF011A_141' '' } %GIDa_f591e2ef_fc9c_4595_adda_387f88e3652b"  Value=EotLrngEotLrnTmr
  wires:
  TmrElpdDetn/1 -> EotCcwLrgnDetd/Action
  Divide2/1 -> Relational Operator1/1  "In MilliSec"
  MillisecPerCount/1 -> Divide2/2
  GetTiSpan100MicroSec32bit/1(TiSpan) -> Divide2/1
  Relational Operator1/1 -> TmrElpdDetn/1
  calibration6/1 -> Relational Operator1/2
  Data Store Read1/1 -> GetTiSpan100MicroSec32bit/1(RefTmr)

== system SF011A_EotLrng/EotLrng/EotLrngPer1/SRLNotEna/LrnEotLim/LrgnEotCmplSts/EotCwElpdTmr ==
  Action Port : ActionPort  ActionType=else
  CopyRight2 : Subsystem  Description=|  mask(Copyright Information){none=on}
      | Copyright info block.                                               
      |                                                                     
      | Place copyright information at the top of every subsystem in design.
      mask prompts: none "No parameters"
      mask help: Place copyright information at the top of every subsystem in design.
      mask Display:
      | NxtrConf = 'Nexteer Confidential';
      | 
      | sys = bdroot; %handle for the current model ("system")
      | first = get_param(sys,'Created');
      | if(isempty(first))
      |     first = datestr(now,'yyyy');
      | else
      |     first = first(end-3:end);  %year is last four digits
      | end
      | 
      | last = get_param(sys,'LastModifiedDate');
      | if isempty(last)
      |     last = datestr(now,'yyyy');
      | else
      |     last = last(end-3:end);
      | end
      | 
      | if strcmp(first,last)
      |     fprintf('%s -- Copyright %s Nexteer',NxtrConf,first)
      | else
      |     fprintf('%s -- %s%s- %s Nexteer',NxtrConf,char(169),first,last)
      | end
  Data Store Read : DataStoreRead  RequirementInfo="{'linktype_rmi_doors' '0000ba59 (/E-STEER Core/SubSystem Specifications/Application Functions/SF011A Learned EOT Limits)' '#SF011A_139' 'true' 'REQ:  SF011A_139' '' } %GIDa_0cbd550f_330c_41bb_a3f2_a3c446e662b1"  DataStoreName=CwEotRefTmr
  Divide2 : Product  RequirementInfo="{'linktype_rmi_doors' '0000ba59 (/E-STEER Core/SubSystem Specifications/Application Functions/SF011A Learned EOT Limits)' '#SF011A_139' 'true' 'REQ:  SF011A_139' '' } %GIDa_136b1c80_3b7a_40f9_a43c_3ae83635ec69"  Inputs=**
  EotCwLrgnDetd : Subsystem  RequirementInfo="{'linktype_rmi_doors' '0000ba59 (/E-STEER Core/SubSystem Specifications/Application Functions/SF011A Learned EOT Limits)' '#SF011A_139' 'true' 'REQ:  SF011A_139' '' } %GIDa_d7a89013_0afc_4478_ba05_072edac54bae"  TreatAsAtomicUnit=on
  GetTiSpan100MicroSec32bit : Subsystem  mask(Timer_GTS){}
      mask help: Used to get the time span between start and current time.
  MillisecPerCount : Constant  RequirementInfo="{'linktype_rmi_doors' '0000ba59 (/E-STEER Core/SubSystem Specifications/Application Functions/SF011A Learned EOT Limits)' '#SF011A_139' 'true' 'REQ:  SF011A_139' '' } %GIDa_add1d887_85cb_46c3_bc7c_09008b28374f"  Value=CNVTOMILLISEC_MILLISECPERCNT_F32
  Relational Operator1 : RelationalOperator  RequirementInfo="{'linktype_rmi_doors' '0000ba59 (/E-STEER Core/SubSystem Specifications/Application Functions/SF011A Learned EOT Limits)' '#SF011A_139' 'true' 'REQ:  SF011A_139' '' } %GIDa_6a37739d_48e2_4b9b_b4f9_2c152969b6d4"  OutDataTypeStr=boolean
  TmrElpdDetn : If  RequirementInfo="{'linktype_rmi_doors' '0000ba59 (/E-STEER Core/SubSystem Specifications/Application Functions/SF011A Learned EOT Limits)' '#SF011A_139' 'true' 'REQ:  SF011A_139' '' } %GIDa_5e06e2bc_f22e_4192_88ff_b5732ffa7091"  IfExpression=u1  ShowElse=off
  calibration5 : Constant  RequirementInfo="{'linktype_rmi_doors' '0000ba59 (/E-STEER Core/SubSystem Specifications/Application Functions/SF011A Learned EOT Limits)' '#SF011A_139' 'true' 'REQ:  SF011A_139' '' } %GIDa_490f8226_12f5_4297_b7ee_6d242d4f04fc"  Value=EotLrngEotLrnTmr
  wires:
  Relational Operator1/1 -> TmrElpdDetn/1
  calibration5/1 -> Relational Operator1/2  "In MilliSec"
  Data Store Read/1 -> GetTiSpan100MicroSec32bit/1(RefTmr)
  GetTiSpan100MicroSec32bit/1(TiSpan) -> Divide2/1
  MillisecPerCount/1 -> Divide2/2
  Divide2/1 -> Relational Operator1/1  "In MilliSec"
  TmrElpdDetn/1 -> EotCwLrgnDetd/Action

== system SF011A_EotLrng/EotLrng/EotLrngPer1/SRLNotEna/LrnEotLim/LrgnEotCmplSts/GetRefTmrEotCcw ==
  Action Port : ActionPort  ActionType=then
  CopyRight2 : Subsystem  Description=|  mask(Copyright Information){none=on}
      | Copyright info block.                                               
      |                                                                     
      | Place copyright information at the top of every subsystem in design.
      mask prompts: none "No parameters"
      mask help: Place copyright information at the top of every subsystem in design.
      mask Display:
      | NxtrConf = 'Nexteer Confidential';
      | 
      | sys = bdroot; %handle for the current model ("system")
      | first = get_param(sys,'Created');
      | if(isempty(first))
      |     first = datestr(now,'yyyy');
      | else
      |     first = first(end-3:end);  %year is last four digits
      | end
      | 
      | last = get_param(sys,'LastModifiedDate');
      | if isempty(last)
      |     last = datestr(now,'yyyy');
      | else
      |     last = last(end-3:end);
      | end
      | 
      | if strcmp(first,last)
      |     fprintf('%s -- Copyright %s Nexteer',NxtrConf,first)
      | else
      |     fprintf('%s -- %s%s- %s Nexteer',NxtrConf,char(169),first,last)
      | end
  Data Store Write2 : DataStoreWrite  RequirementInfo={} %GIDa_bbd062ed_8377_403f_a800_c7deb734e0cd  DataStoreName=CcwEotRefTmr
  GetRefTmr100MicroSec32bit1 : Subsystem  RequirementInfo={} %GIDa_62693dee_9fea_406d_81e7_cde3ad5fb2b9
  wires:
  GetRefTmr100MicroSec32bit1/1(RefTmr) -> Data Store Write2/1

== system SF011A_EotLrng/EotLrng/EotLrngPer1/SRLNotEna/LrnEotLim/LrgnEotCmplSts/GetRefTmrEotCw ==
  Action Port : ActionPort  ActionType=then
  CopyRight2 : Subsystem  Description=|  mask(Copyright Information){none=on}
      | Copyright info block.                                               
      |                                                                     
      | Place copyright information at the top of every subsystem in design.
      mask prompts: none "No parameters"
      mask help: Place copyright information at the top of every subsystem in design.
      mask Display:
      | NxtrConf = 'Nexteer Confidential';
      | 
      | sys = bdroot; %handle for the current model ("system")
      | first = get_param(sys,'Created');
      | if(isempty(first))
      |     first = datestr(now,'yyyy');
      | else
      |     first = first(end-3:end);  %year is last four digits
      | end
      | 
      | last = get_param(sys,'LastModifiedDate');
      | if isempty(last)
      |     last = datestr(now,'yyyy');
      | else
      |     last = last(end-3:end);
      | end
      | 
      | if strcmp(first,last)
      |     fprintf('%s -- Copyright %s Nexteer',NxtrConf,first)
      | else
      |     fprintf('%s -- %s%s- %s Nexteer',NxtrConf,char(169),first,last)
      | end
  Data Store Write1 : DataStoreWrite  RequirementInfo={} %GIDa_5ab0b6ec_8b77_4411_bea3_55d98c476632  DataStoreName=CwEotRefTmr
  GetRefTmr100MicroSec32bit : Subsystem  RequirementInfo={} %GIDa_14016f36_76c6_4aab_9bb2_1b7244b9ba42
  wires:
  GetRefTmr100MicroSec32bit/1(RefTmr) -> Data Store Write1/1
